simulink model "ansiOct"  (R2018a)
settings: Solver=VariableStepAuto  StartTime=0.0  StopTime=0.1  RelTol=1e-3
undefined symbols (not defined in the file or in its folder): fdesignblkfcn, G1, G2, G3, G4, G5, G6, G7, G8, gcbh, get, T
libraries: dspsrcs4 x1, dspxfrm3 x1, dspobslib x1
(part 1 of 4)
settings Model: Creator=Daniel  LastModifiedBy=Daniel

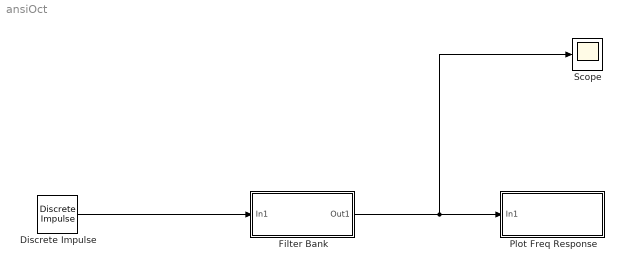
== system ansiOct ==
  Discrete Impulse : dspsrcs4/Discrete  Impulse  Delay=0  SampleTime=T  FrameSample=128  OutputFrames=off  dataType=double  isSigned=on  wordLen=16  udDataType=sfix(16)  fracBitsMode=Best precision  numFracBits=15  OutDataTypeStr=double  LastOutDataTypeStr=double
  "Filter Bank " : Subsystem
  Plot Freq Response : Subsystem
  Scope : Scope
  wires:
  "Filter Bank "/1(Out1) -> Scope/1, Plot Freq Response/1(In1)
  Discrete Impulse/1 -> "Filter Bank "/1(In1)

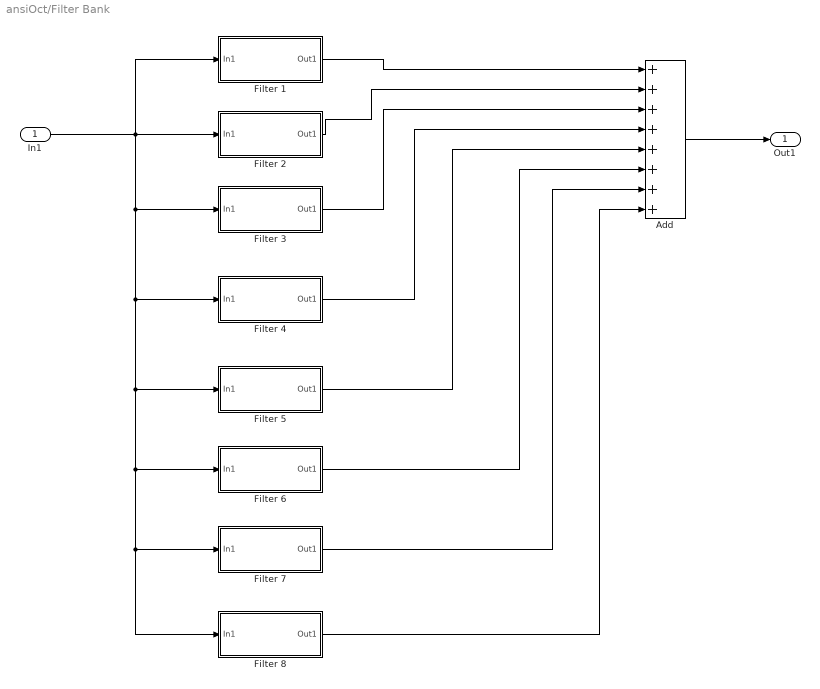
== system ansiOct/Filter Bank  ==
  In1 : Inport
  Add : Sum  Inputs=++++++++
  Filter 1 : Subsystem
  Filter 2 : Subsystem
  Filter 3 : Subsystem
  Filter 4 : Subsystem
  Filter 5 : Subsystem
  Filter 6 : Subsystem
  Filter 7 : Subsystem
  Filter 8 : Subsystem
  Out1 : Outport
  wires:
  In1/1 -> Filter 6/1(In1), Filter 8/1(In1), Filter 7/1(In1), Filter 5/1(In1), Filter 4/1(In1), Filter 3/1(In1), Filter 1/1(In1), Filter 2/1(In1)
  Add/1 -> Out1/1
  Filter 1/1(Out1) -> Add/1
  Filter 2/1(Out1) -> Add/2
  Filter 3/1(Out1) -> Add/3
  Filter 4/1(Out1) -> Add/4
  Filter 5/1(Out1) -> Add/5
  Filter 6/1(Out1) -> Add/6
  Filter 7/1(Out1) -> Add/7
  Filter 8/1(Out1) -> Add/8

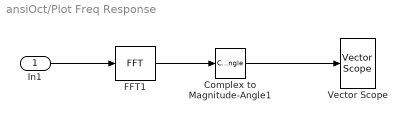
== system ansiOct/Plot Freq Response ==
  In1 : Inport
  Complex to Magnitude-Angle1 : ComplexToMagnitudeAngle  Output=Magnitude
  FFT1 : dspxfrm3/FFT  FFTImplementation=Auto  CompMethod=Table lookup  TableOpt=NEW  TableOptActive=Speed  BitRevOrder=off  Normalize=off  InheritFFTLength=on  FFTLength=64  WrapInput=on  roundingMode=Floor  overflowMode=off  firstCoeffDataTypeStr=Inherit: Same word length as input  firstCoeffLastDataTypeStr=Inherit: Same word length as input  outputMin=[]  outputMax=[]
  Vector Scope : dspobslib/Vector Scope  ScopeProperties=off  Domain=Frequency  HorizSpan=1  DisplayProperties=off  AxisGrid=on  Memory=off  FrameNumber=off  AxisLegend=off  AxisZoom=off  OpenScopeAtSimStart=on  OpenScopeImmediately=off  FigPos=get(0,'defaultfigureposition')  AxisProperties=on  XUnits=Hertz  XRange=[0...Fs/2]  InheritXIncr=on  XIncr=1  XLabel=Samples  XLimit=Auto  XMin=0  XMax=1  XStart=0  YUnits=dB  YLabel=|Magnitude (dB)|  LineProperties=off  XAxisParamsVer=6.9
      settings: SourceProductName=DSP System Toolbox  SourceProductBaseCode=DS  YMin=0.0723692553519949  YMax=69.3188381671759
  wires:
  In1/1 -> FFT1/1
  FFT1/1 -> Complex to Magnitude-Angle1/1
  Complex to Magnitude-Angle1/1 -> Vector Scope/1

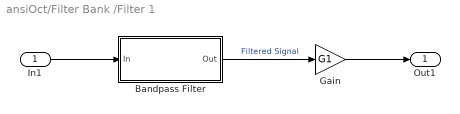
== system ansiOct/Filter Bank /Filter 1 ==
  In1 : Inport
  Bandpass Filter : Subsystem  DialogController=fdesignblkfcn  InitFcn=fdesignblkfcn(gcbh, {'InitFcn'});  mask(Bandpass Filter){}
      mask help: Design a bandpass filter
      settings: CopyFcn=fdesignblkfcn(gcbh, {'CopyFcn'});
      mask Help: helpview(mapfilelocation('dsp'), 'dspbandpassfilter');
      mask Display: disp('Bandpass');
  Gain : Gain  Gain=G1
  Out1 : Outport
  wires:
  Bandpass Filter/1(Out) -> Gain/1  "Filtered Signal"
  In1/1 -> Bandpass Filter/1(In)
  Gain/1 -> Out1/1

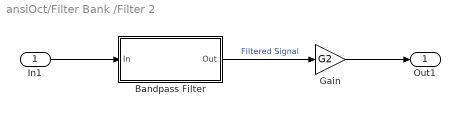
== system ansiOct/Filter Bank /Filter 2 ==
  In1 : Inport
  Bandpass Filter : Subsystem  DialogController=fdesignblkfcn  InitFcn=fdesignblkfcn(gcbh, {'InitFcn'});  mask(Bandpass Filter){}
      mask help: Design a bandpass filter
      settings: CopyFcn=fdesignblkfcn(gcbh, {'CopyFcn'});
      mask Help: helpview(mapfilelocation('dsp'), 'dspbandpassfilter');
      mask Display: disp('Bandpass');
  Gain : Gain  Gain=G2
  Out1 : Outport
  wires:
  Bandpass Filter/1(Out) -> Gain/1  "Filtered Signal"
  In1/1 -> Bandpass Filter/1(In)
  Gain/1 -> Out1/1

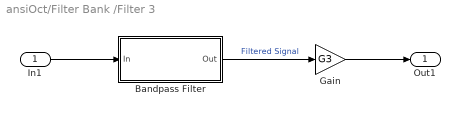
== system ansiOct/Filter Bank /Filter 3 ==
  In1 : Inport
  Bandpass Filter : Subsystem  DialogController=fdesignblkfcn  InitFcn=fdesignblkfcn(gcbh, {'InitFcn'});  mask(Bandpass Filter){}
      mask help: Design a bandpass filter
      settings: CopyFcn=fdesignblkfcn(gcbh, {'CopyFcn'});
      mask Help: helpview(mapfilelocation('dsp'), 'dspbandpassfilter');
      mask Display: disp('Bandpass');
  Gain : Gain  Gain=G3
  Out1 : Outport
  wires:
  Bandpass Filter/1(Out) -> Gain/1  "Filtered Signal"
  In1/1 -> Bandpass Filter/1(In)
  Gain/1 -> Out1/1

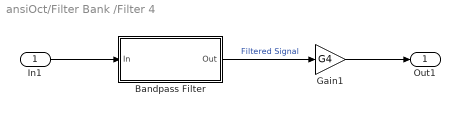
== system ansiOct/Filter Bank /Filter 4 ==
  In1 : Inport
  Bandpass Filter : Subsystem  DialogController=fdesignblkfcn  InitFcn=fdesignblkfcn(gcbh, {'InitFcn'});  mask(Bandpass Filter){}
      mask help: Design a bandpass filter
      settings: CopyFcn=fdesignblkfcn(gcbh, {'CopyFcn'});
      mask Help: helpview(mapfilelocation('dsp'), 'dspbandpassfilter');
      mask Display: disp('Bandpass');
  Gain1 : Gain  Gain=G4
  Out1 : Outport
  wires:
  Bandpass Filter/1(Out) -> Gain1/1  "Filtered Signal"
  In1/1 -> Bandpass Filter/1(In)
  Gain1/1 -> Out1/1

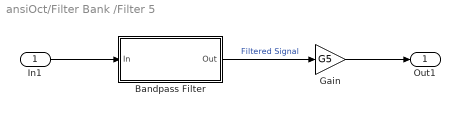
== system ansiOct/Filter Bank /Filter 5 ==
  In1 : Inport
  Bandpass Filter : Subsystem  DialogController=fdesignblkfcn  InitFcn=fdesignblkfcn(gcbh, {'InitFcn'});  mask(Bandpass Filter){}
      mask help: Design a bandpass filter
      settings: CopyFcn=fdesignblkfcn(gcbh, {'CopyFcn'});
      mask Help: helpview(mapfilelocation('dsp'), 'dspbandpassfilter');
      mask Display: disp('Bandpass');
  Gain : Gain  Gain=G5
  Out1 : Outport
  wires:
  Bandpass Filter/1(Out) -> Gain/1  "Filtered Signal"
  In1/1 -> Bandpass Filter/1(In)
  Gain/1 -> Out1/1

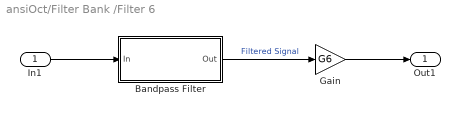
== system ansiOct/Filter Bank /Filter 6 ==
  In1 : Inport
  Bandpass Filter : Subsystem  DialogController=fdesignblkfcn  InitFcn=fdesignblkfcn(gcbh, {'InitFcn'});  mask(Bandpass Filter){}
      mask help: Design a bandpass filter
      settings: CopyFcn=fdesignblkfcn(gcbh, {'CopyFcn'});
      mask Help: helpview(mapfilelocation('dsp'), 'dspbandpassfilter');
      mask Display: disp('Bandpass');
  Gain : Gain  Gain=G6
  Out1 : Outport
  wires:
  Bandpass Filter/1(Out) -> Gain/1  "Filtered Signal"
  In1/1 -> Bandpass Filter/1(In)
  Gain/1 -> Out1/1

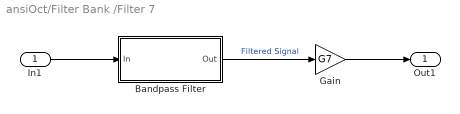
== system ansiOct/Filter Bank /Filter 7 ==
  In1 : Inport
  Bandpass Filter : Subsystem  DialogController=fdesignblkfcn  InitFcn=fdesignblkfcn(gcbh, {'InitFcn'});  mask(Bandpass Filter){}
      mask help: Design a bandpass filter
      settings: CopyFcn=fdesignblkfcn(gcbh, {'CopyFcn'});
      mask Help: helpview(mapfilelocation('dsp'), 'dspbandpassfilter');
      mask Display: disp('Bandpass');
  Gain : Gain  Gain=G7
  Out1 : Outport
  wires:
  Bandpass Filter/1(Out) -> Gain/1  "Filtered Signal"
  In1/1 -> Bandpass Filter/1(In)
  Gain/1 -> Out1/1

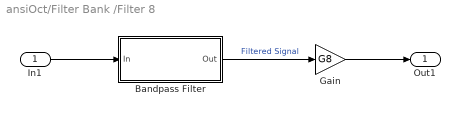
== system ansiOct/Filter Bank /Filter 8 ==
  In1 : Inport
  Bandpass Filter : Subsystem  DialogController=fdesignblkfcn  InitFcn=fdesignblkfcn(gcbh, {'InitFcn'});  mask(Bandpass Filter){}
      mask help: Design a bandpass filter
      settings: CopyFcn=fdesignblkfcn(gcbh, {'CopyFcn'});
      mask Help: helpview(mapfilelocation('dsp'), 'dspbandpassfilter');
      mask Display: disp('Bandpass');
  Gain : Gain  Gain=G8
  Out1 : Outport
  wires:
  Bandpass Filter/1(Out) -> Gain/1  "Filtered Signal"
  In1/1 -> Bandpass Filter/1(In)
  Gain/1 -> Out1/1

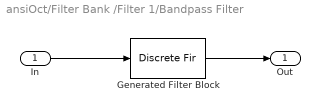
== system ansiOct/Filter Bank /Filter 1/Bandpass Filter ==
  In : Inport
  Generated Filter Block : DiscreteFir  Tag=BlockMethodSubSystem  Coefficients=[-0.00766321048125649575 -0.000180280651799153227 -0.000182785610599459888 -0.000184443947717255431 -0.000186875509306509973 -0.000188447846206871888 -0.000190806976946802253 -0.000192297232951844953 -0.000194601991788270897 -0.00019601436629961916 -0.000198275924662991339 -0.000199627261288770776 -0.000201883607460546632 -0.000203184800043465665 -0.000205446856650040425 -0.00020671435309735123 -0.000209021020418383147 -0.000210261818703512887 -0.000212637221751146529 -0.000213844970491127952 -0.000216312251259223495 -0.000217446489720575498 -0.000219982388833387494 -0.000220951767083763553 -0.000223524562204970441 -0.000224120349799630114 -0.000226602607415899191 -0.000226381163353264617 -0.00022855196562423567 -0.000226411808115840803 -0.00022788720417254318 -0.000218210628464381948 -0.00023497568852827173 -0.000235388195940166792 -0.000231911709631520764 -0.000234847237306085694 -0.000234218286249015877 -0.000236191010248064457 -0.000236133326835806843 -0.000237658198580002181 -0.000237824374138780997 -0.000239065536242846706 -0.000239314711244092911 -0.000240322217095325909 -0.000240591141967531739 -0.000241395290724512595 -0.000241620289729746522 -0.000242205126466383863 -0.000242348430135221174 -0.000242703332043400462 -0.000242737525589365382 -0.000242852706930902541 -0.000242787694884182074 -0.000242697013428466778 -0.000242571666528661276 -0.000242324138280899378 -0.000242267308889479183 -0.000241981617919248673 -0.000242174795828776633 -0.000241928235265721677 -0.000242552799506668028 -0.000242070080761058314 -0.000242951008045991538 -0.000238837783462793953 -0.000238524395754581635 -0.000240482695051520088 -0.000238131971158704278 -0.000238361412433516894 -0.000236819695529160888 -0.000236560261147229436 -0.000235120745499842995 -0.000234566442548079878 -0.000233107877824311778 -0.000232337262237553173 -0.000230824115358478572 -0.000229864201716600055 -0.000228284338687220778 -0.000227186908550826142 -0.000225559522026170975 -0.000224348391177660712 -0.000222687157823483751 -0.000221384895594229806 -0.000219695252986035498 -0.000218288750798940076 -0.000216538362972683925 -0.000215001242463077377 -0.000213138473820173368 -0.00021137502997300566 -0.00020932487579477152 -0.000207285265296331268 -0.000205074486160273492 -0.000202836270805567716 -0.000200765041235944123 -0.0001987055480711205 -0.000197532405615366671 -0.000195150188842548315 -0.000191209642438303908 -0.000190276841143980876 -0.000187202487362218481 -0.000185240501569416515 -0.000182390551951532839 -0.000180230839448019208 -0.000177405086298491356 -0.000175124754402528754 -0.000172279163601710529 -0.00016990718351105356 -0.000167034234510909918 -0.0001645707226866152 -0.000161631089549796341 -0.000159065166646553364 -0.000156051458345740201 -0.000153373891334594725 -0.000150275575470940439 -0.000147492921320956853 -0.000144332775467802981 -0.000141480139864228469 -0.000138283780954060647 -0.000135415111981151 -0.000132253194449095615 -0.00012939794160146811 -0.00012624810089431344 -0.000123340216162112239 -0.000120087655605361277 -0.000116953606323112299 -0.000113461213084915954 -0.000110146192055487669 -0.000107019722237994779 -0.000104842362745944295 -0.000100502507666445714 -9.78003219176787851e-05 -9.4336203158837246e-05 -9.12975976423785826e-05 -8.78539591674525901e-05 -8.47643640689416643e-05 -8.13133957190324786e-05 -7.81920543152074147e-05 -7.47265782922943702e-05 -7.15827263485615043e-05 -6.81264144678822337e-05 -6.49982664947454912e-05 -6.15649773568770117e-05 -5.84607907311234548e-05 -5.50704538519423354e-05 -5.20035077315376368e-05 -4.86539618035929832e-05 -4.56102787262149857e-05 -4.2282737317105895e-05 -3.92543763503132596e-05 -3.59172242501717447e-05 -3.28782288113433865e-05 -2.95601830281163969e-05 -2.65807669006965147e-05 -2.33565234231638626e-05 -2.05227470835534791e-05 -1.74520927754650633e-05 -1.4738187019845262e-05 -1.16039801579321895e-05 -8.66918652024433953e-06 -5.19344793675175057e-06 -3.17781433741570398e-06 ...(+28602 chars)]  InputProcessing=Columns as channels (frame based)
  Out : Outport
  wires:
  In/1 -> Generated Filter Block/1
  Generated Filter Block/1 -> Out/1
